simulink model "asymmetricPwm"  (R2021a)
settings: Solver=FixedStepAuto  StartTime=0.0  StopTime=10.0  RelTol=1e-3
settings Model: Creator=Z634594  LastModifiedBy=Z634594

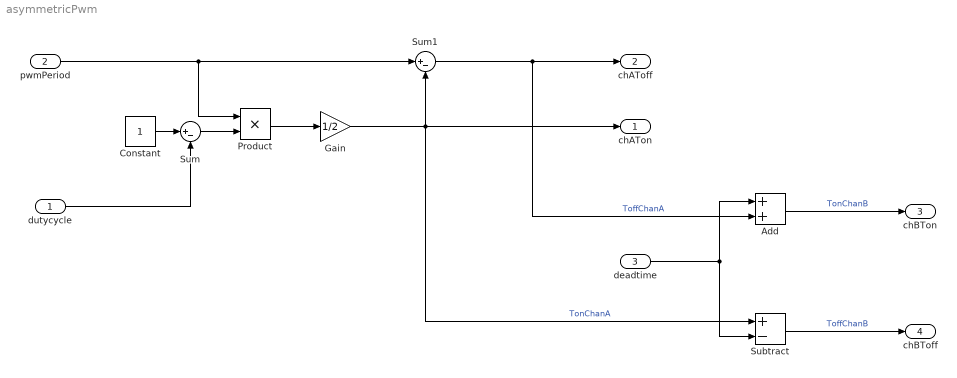
== system asymmetricPwm ==
  dutycycle : Inport  PortDimensions=3
  pwmPeriod : Inport  Port=2
  deadtime : Inport  Port=3
  Add : Sum
  Constant : Constant
  Gain : Gain  Gain=1/2
  Product : Product
  Subtract : Sum  Inputs=+-
  Sum : Sum  Inputs=|+-
  Sum1 : Sum  Inputs=|+-
  chATon : Outport  PortDimensions=3
  chAToff : Outport  Port=2  PortDimensions=3
  chBTon : Outport  Port=3  PortDimensions=3
  chBToff : Outport  Port=4  PortDimensions=3
  wires:
  Add/1 -> chBTon/1  "TonChanB"
  Constant/1 -> Sum/1
  Gain/1 -> chATon/1, Subtract/1, Sum1/2  "TonChanA"
  Product/1 -> Gain/1
  Subtract/1 -> chBToff/1  "ToffChanB"
  Sum1/1 -> Add/2, chAToff/1  "ToffChanA"
  deadtime/1 -> Add/1, Subtract/2
  dutycycle/1 -> Sum/2
  Sum/1 -> Product/2
  pwmPeriod/1 -> Sum1/1, Product/1
